simulink library "lib_methods"  (Simulink 7.7)
settings: Solver=ode45  StartTime=0.0  StopTime=10.0  RelTol=1e-3
undefined symbols (not defined in the file): AOBC_dt, DiscIntNeverNeededParam, dt, I, mom_lim, MTQ_out, Ratelim, RW_J, target_mom, three_one_skew_matrix, UT1_UTC
libraries: aerolibutil x15, lib_util x15, vrlib x4, lib_astrodynamics x3, aerolibtransform2 x1, lib_methods x1, lib_env x1
(part 2 of 2)

== matlab function attitude determination/UDUpdate ==
  data: UP input double; UP1 output double; DP1 output double; DP input double; UQ input double; DQ input double; PHI input double; x input double; x1 output double; H input double; R input double; y input double; ObsUpdate input double
function [UP1, DP1,x1] = UDUpdate(UP,DP,UQ,DQ,PHI,x,H,R,y,ObsUpdate)
%#codegen

W = [PHI * UP UQ];

[nDProw,nDPcol] = size(DP);
[nDQrow,nDQcol] = size(DQ);

zero1 = zeros(nDProw, nDQcol);
zero2 = zeros(nDQrow, nDPcol);

F = [DP zero1; zero2 DQ];

[nWrow,nWcol] = size(W);

for j = nWrow:-1:2
    v = W(j,:);
    z = v * F;
    
    temp = z * v';
    DP(j,j) = temp(1,1);
    for i = 1:j
        temp = W(i,:);
        temp2 = temp * z';
        UP(i,j) = temp2(1,1) / DP(j,j);
        W(i,:) = W(i,:) - UP(i,j) * v;
    end
end

temp = W(1,:);
temp2 = temp * F * temp';
DP(1,1) = temp2(1,1);

UP1 = UP;
DP1 = DP;
x1 = PHI * x;

if ObsUpdate > 0.5

    U = UP1;
    D = DP1;
    x = x1;
    
    [nUrow,nUcol] = size(U);
    
    for i = 1:nUrow
        U(i,i) = D(i,i);
    end

    [nHrow,nHcol] = size(H);

    FF = zeros(nHcol,1);
    GG = zeros(nHcol,1);

    for L = 1:nHrow
        y(L) = y(L) - H(L,:) * x;
        
        for j = nHcol:-1:2
            FF(j) = H(L,j) + H(L,1:j-1) * U(1:j-1,j);
            GG(j) = U(j,j) * FF(j);
        end
        
        FF(1) = H(L,1);
        GG(1) = U(1,1) * FF(1);
        alpha = R(L,L) + FF(1) * GG(1);
        gamma = 1 / alpha;
        U(1,1) = R(L,L) * gamma * U(1,1);

        for j = 2:nHcol
            beta = alpha;
            alpha = alpha + FF(j) * GG(j);
            lambda = FF(j) * gamma;
            gamma = 1 / alpha;
            U(j,j) = beta * U(j,j) * gamma;
            beta = U(1:j-1,j);

            U(1:j-1,j) = beta - lambda * GG(1:j-1);
            GG(1:j-1) = GG(1:j-1) + GG(j) * beta;
        end
        y(L) = y(L) * gamma;
        x = x + GG * y(L);
    end

    DP1 = D;
    UP1 = U;
    x1 = x;
    
    for i = 1:nUrow
        DP1(i,i) = U(i,i);
        UP1(i,i) = 1.0;
    end
    
end

== matlab function attitude determination/UDdecomp1 ==
  data: P input double; U output double; D output double
function [U, D] = UDdecomposition(P)
%#codegen

[nProw, nPcol] = size(P);

U = zeros(nProw);
D = zeros(nProw);

for k = nProw:-1:2
    D(k,k) = P(k,k);
    U(k,k) = 1.0;
    for j = 1:k-1
        U(j,k) = P(j,k) / D(k,k);
        for i = 1:j
            P(i,j) = P(i,j) - U(i,k) * U(j,k) * D(k,k);
        end
    end
end

U(1,1) = 1.0;
D(1,1) = P(1,1);

== matlab function attitude determination/Uinv ==
  data: U input double; Uinv output double
function Uinv = Uinverse(U)
%#codegen

[nUrow, nUcol] = size(U);

Uinv = zeros(nUrow);

for i = 1:nUrow
for j = 1:nUrow
    if i > j
        Uinv(i,j) = 0.0;
    elseif i == j
        Uinv(i,j) = 1.0 / U(i,j);
    else
        sum = 0.0;
        for k = i:j-1
            sum = sum + Uinv(i,k) * U(k,j);
        end
        Uinv(i,j) = -sum / U(j,j);
    end
end
end

== matlab function attitude determination/calc PHI ==
  data: w input double; PHI output double; dt input double
function PHI = fcn(w, dt)
%#codegen

F = [    0  w(3) -w(2)  -0.5     0     0; ...
     -w(3)     0  w(1)     0  -0.5     0; ...
      w(2) -w(1)     0     0     0  -0.5; ...
         0     0     0     0     0     0; ...
         0     0     0     0     0     0; ...
         0     0     0     0     0     0];
% F = [    0  0.0 0.0   -0.5     0     0; ...
%      0 0 0     0   -0.5     0; ...
%       0 0     0     0     0   -0.5; ...
%          0     0     0     0     0     0; ...
%          0     0     0     0     0     0; ...
%          0     0     0     0     0     0];
    
I = eye(size(F));

PHI = I + F * dt + F^2 * dt^2 / 2 + F^3 * dt^3 / 6.0 + F^4 * dt^4 / 24.0;

== matlab function attitude determination/dynamics ==
  data: q input double; rate input double; d_q output double
function d_q  = att_dyn(q, rate)

%#codegen

% dq/dt = 1/2 * [    0      -rate'] * q
%               [ rate -rate_tilde] 
d_q = 0.5 * [       0 -rate(1) -rate(2) -rate(3);...
              rate(1)        0  rate(3) -rate(2);...
              rate(2) -rate(3)       0   rate(1);...
              rate(3)  rate(2) -rate(1)        0] * q;

== matlab function attitude determination/dynamics1 ==
  data: q input double; rate input double; d_q output double
function d_q  = att_dyn(q, rate)

%#codegen

% dq/dt = 1/2 * [    0      -rate'] * q
%               [ rate -rate_tilde] 
d_q = 0.5 * [       0 -rate(1) -rate(2) -rate(3);...
              rate(1)        0  rate(3) -rate(2);...
              rate(2) -rate(3)       0   rate(1);...
              rate(3)  rate(2) -rate(1)        0] * q;

== matlab function coarse kalman/UDUpdate ==
  data: UP input double; UP1 output double; DP1 output double; DP input double; UQ input double; DQ input double; PHI input double; x input double; x1 output double; H input double; R input double; y input double; ObsUpdate input double
function [UP1, DP1,x1] = UDUpdate(UP,DP,UQ,DQ,PHI,x,H,R,y,ObsUpdate)
%#codegen

W = [PHI * UP UQ];

[nDProw,nDPcol] = size(DP);
[nDQrow,nDQcol] = size(DQ);

zero1 = zeros(nDProw, nDQcol);
zero2 = zeros(nDQrow, nDPcol);

F = [DP zero1; zero2 DQ];

[nWrow,nWcol] = size(W);

for j = nWrow:-1:2
    v = W(j,:);
    z = v * F;
    
    temp = z * v';
    DP(j,j) = temp(1,1);
    for i = 1:j
        temp = W(i,:);
        temp2 = temp * z';
        UP(i,j) = temp2(1,1) / DP(j,j);
        W(i,:) = W(i,:) - UP(i,j) * v;
    end
end

temp = W(1,:);
temp2 = temp * F * temp';
DP(1,1) = temp2(1,1);

UP1 = UP;
DP1 = DP;
x1 = PHI * x;

if ObsUpdate > 0.5

    U = UP1;
    D = DP1;
    x = x1;
    
    [nUrow,nUcol] = size(U);
    
    for i = 1:nUrow
        U(i,i) = D(i,i);
    end

    [nHrow,nHcol] = size(H);

    FF = zeros(nHcol,1);
    GG = zeros(nHcol,1);

    for L = 1:nHrow
        y(L) = y(L) - H(L,:) * x;
        
        for j = nHcol:-1:2
            FF(j) = H(L,j) + H(L,1:j-1) * U(1:j-1,j);
            GG(j) = U(j,j) * FF(j);
        end
        
        FF(1) = H(L,1);
        GG(1) = U(1,1) * FF(1);
        alpha = R(L,L) + FF(1) * GG(1);
        gamma = 1 / alpha;
        U(1,1) = R(L,L) * gamma * U(1,1);

        for j = 2:nHcol
            beta = alpha;
            alpha = alpha + FF(j) * GG(j);
            lambda = FF(j) * gamma;
            gamma = 1 / alpha;
            U(j,j) = beta * U(j,j) * gamma;
            beta = U(1:j-1,j);

            U(1:j-1,j) = beta - lambda * GG(1:j-1);
            GG(1:j-1) = GG(1:j-1) + GG(j) * beta;
        end
        y(L) = y(L) * gamma;
        x = x + GG * y(L);
    end

    DP1 = D;
    UP1 = U;
    x1 = x;
    
    for i = 1:nUrow
        DP1(i,i) = U(i,i);
        UP1(i,i) = 1.0;
    end
    
end

== matlab function coarse kalman/UDdecomp1 ==
  data: P input double; U output double; D output double
function [U, D] = UDdecomposition(P)
%#codegen

[nProw, nPcol] = size(P);

U = zeros(nProw);
D = zeros(nProw);

for k = nProw:-1:2
    D(k,k) = P(k,k);
    U(k,k) = 1.0;
    for j = 1:k-1
        U(j,k) = P(j,k) / D(k,k);
        for i = 1:j
            P(i,j) = P(i,j) - U(i,k) * U(j,k) * D(k,k);
        end
    end
end

U(1,1) = 1.0;
D(1,1) = P(1,1);

== matlab function q_method ==
  data: r1_i input double; y output double; r2_i input double; r1_b input double; r2_b input double
function y  = fcn(r1_i, r2_i, r1_b, r2_b)
%#codegen

r1_i = r1_i / norm(r1_i);
r2_i = r2_i / norm(r2_i);
r1_b = r1_b / norm(r1_b);
r2_b = r2_b / norm(r2_b);

a1 = 0.99;
a2 = 0.01;

B = a1 * r1_b * r1_i' + a2 * r2_b * r2_i';
sigma = trace(B);
S = B + B';
z = a1 * cross(r1_b, r1_i) + a2 * cross(r2_b, r2_i);

I = eye(3);

%K = [S(1,1) - sigma, S(1,2), S(1,3), z(1);
%     S(2,1), S(2,2) - sigma, S(2,3), z(2);
%     S(3,1), S(3,2), S(3,3) - sigma, z(3);
%     z(1), z(2), z(3), sigma];

K = [sigma, z';
     z, S - sigma * I];

[V,D] = eig(K);
%y=D;
max = -1;
maxi = 0;
for i = 1:4
    if max < real(D(i,i))
        max = real(D(i,i));
        maxi = i;
    end
end
%y = maxi;
y = [real(V(1,maxi)) real(V(2,maxi)) real(V(3,maxi)) real(V(4,maxi))];

== matlab function calc earth pointing/MATLAB Function2 ==
  data: R input double; nd output double; V input double
function nd = fcn(R,V)
%#codegen

normR = norm(R);

nd = (-V * normR + R * (R' * V) / normR) / normR^2;

== matlab function orbit determination/MATLAB Function1 ==
  data: RV input double; OE output double
function OE = OEfcn(RV)
%#codegen

GE = 3.986004415e+5; % km^3/s^2

r = [RV(1); RV(2); RV(3)];
v = [RV(4); RV(5); RV(6)];
r_norm = sqrt(r(1)^2 + r(2)^2 + r(3)^2);
v_norm = sqrt(v(1)^2 + v(2)^2 + v(3)^2);

h = cross(r, v);
h_norm = sqrt(h(1)^2 + h(2)^2 + h(3)^2);

z = [0; 0; 1];
n = cross(z, h);
n_norm = sqrt(n(1)^2 + n(2)^2 + n(3)^2);

e = ((v_norm^2 - GE / r_norm) * r - (r' * v) * v) / GE;
e_norm = sqrt(e(1)^2 + e(2)^2 + e(3)^2);

gsi = v_norm^2 / 2.0 - GE / r_norm;

a = -GE / 2.0 / gsi;

if abs(h(3) / h_norm) > 1
    i = 9999;
else
    i = acos(h(3) / h_norm);
end

if abs(n(1) / n_norm) > 1
    W = 9999;
else
    W = acos(n(1) / n_norm);
end

if abs((n' * e) / n_norm / e_norm) > 1
    w = 9999;
else
    w = acos((n' * e) / n_norm / e_norm);
end

if abs((e' * r) / e_norm / r_norm) > 1
    th = 9999;
else
    th = acos((e' * r) / e_norm / r_norm);
end

if n(2) < 0
    W = 2.0 * pi - W;
end

if e(3) < 0
    w = 2.0 * pi - w;
end

if r' * v < 0
    th = 2.0 * pi - th;
end

if 1.0 - e_norm^2 < 0
    E = 9999;
else
    E = atan2(sin(th) * sqrt(1.0 - e_norm^2), e_norm + cos(th));
end

M = E - e_norm * sin(E);

OE = [a e_norm W i w M];

== matlab function orbit determination/M2th ==
  data: OE input double; W output double; i output double; u output double
function [W,i,u] = OEfcn(OE)
%#codegen

a = OE(1);
e = OE(2);
W = OE(3);
i = OE(4);
w = OE(5);
M = OE(6);

E = 0;

if e < 0.1
    E = M;
    fE  = E - e * sin(E) - M;
    fdE = 1.0 - e * cos(E);
    dE = -fE / fdE;
    E = E + dE;

    while abs(dE) > 1.0e-10
        fE  = E - e * sin(E) - M;
        fdE = 1.0 - e * cos(E);
        dE = -fE / fdE;
        E = E + dE;
    end
    
    th = atan2(sqrt(1.0 - e^2) * sin(E), cos(E) - e);
else
    th = 0;
end

u = w + th;

if e > 1
    e = 0.9;
end
if e < -1
    e = -0.9;
end
